simulink model "requirements"  (R2022a)
settings: Solver=VariableStepAuto  StartTime=0.0  StopTime=10.0  RelTol=1e-3
settings Model: Creator=aldra  LastModifiedBy=aldra
settings ModelReferenceCC: EnableRefExpFcnMdlSchedulingChecks=off
settings RTWCC: Description=Generic Real-Time Target

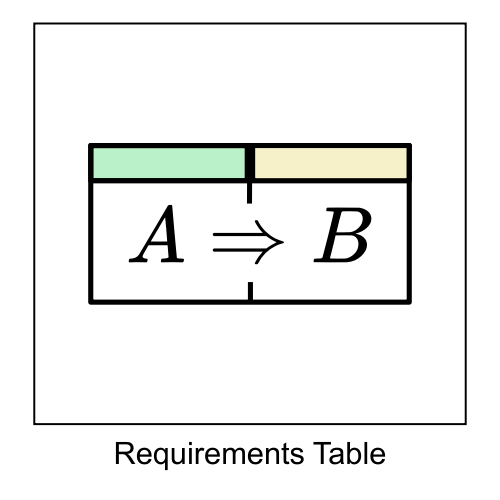
[thumbnail: Simulink's stored preview of the top-level diagram]
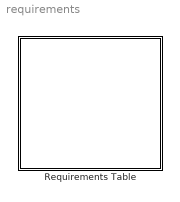
== system requirements ==
  Requirements Table : Requirements Table  TreatAsAtomicUnit=on

== stateflow chart requirements/Requirements Table ==
  (default) -> (junction 1073742735)
  (junction 1073742735) -> (junction 1073742736) : {
      | % SF_REQ_REV_07
      | }
  (junction 1073742736) -> (junction 1073742738) : {
      | % HEADER_ASSIGNMENTS
      |
      | }
  (junction 1073742738) -> (junction 1073742740) : {
      | % START_A_4
      | }
  (junction 1073742740) -> (junction 1073742742) : {
      | }
  (junction 1073742742) -> (junction 1073742744)
  (junction 1073742744) -> (junction 1073742746) : {
      | }
  (junction 1073742746) -> (junction 1073742748) : {
      | % END_A_4
      | }
  (junction 1073742748) -> (junction 1073742750) : {
      | % START_R_1
      | }
  (junction 1073742750) -> (junction 1073742752) : {
      | }
  (junction 1073742752) -> (junction 1073742754) : {
      |
      |
      | }
  (junction 1073742754) -> (junction 1073742756) : {
      | }
  (junction 1073742756) -> (junction 1073742758) : {
      | % START_R_7
      | }
  (junction 1073742758) -> (junction 1073742760) : {
      | }
  (junction 1073742760) -> (junction 1073742762)
  (junction 1073742762) -> (junction 1073742764) [order 1] : [(MODE.AOO == MODE)]
  (junction 1073742762) -> (junction 1073742770) [order 2]
  (junction 1073742764) -> (junction 1073742766) : {
      | reqtable_postcondition((USE_ATR_AMP == true), 'R:1.1');
      |
      |
      | }
  (junction 1073742766) -> (junction 1073742768) : {
      | }
  (junction 1073742768) -> (junction 1073742770)
  (junction 1073742770) -> (junction 1073742772)
  (junction 1073742772) -> (junction 1073742774) : {
      | % END_R_7
      | }
  (junction 1073742774) -> (junction 1073742776) : {
      | % START_R_10
      | }
  (junction 1073742776) -> (junction 1073742778) : {
      | }
  (junction 1073742778) -> (junction 1073742780)
  (junction 1073742780) -> (junction 1073742782) [order 1] : [(MODE.AOO == MODE)]
  (junction 1073742780) -> (junction 1073742788) [order 2]
  (junction 1073742782) -> (junction 1073742784) : {
      | reqtable_postcondition((OUTPUT_ATR == true), 'R:1.2');
      |
      |
      | }
  (junction 1073742784) -> (junction 1073742786) : {
      | }
  (junction 1073742786) -> (junction 1073742788)
  (junction 1073742788) -> (junction 1073742790)
  (junction 1073742790) -> (junction 1073742792) : {
      | % END_R_10
      | }
  (junction 1073742792) -> (junction 1073742794) : {
      | % START_R_40
      | }
  (junction 1073742794) -> (junction 1073742796) : {
      | }
  (junction 1073742796) -> (junction 1073742798) : {
      |
      |
      | }
  (junction 1073742798) -> (junction 1073742800) : {
      | }
  (junction 1073742800) -> (junction 1073742802) : {
      | % START_R_43
      | }
  (junction 1073742802) -> (junction 1073742804) : {
      | }
  (junction 1073742804) -> (junction 1073742806)
  (junction 1073742806) -> (junction 1073742808) [order 1] : [(DISCHARGE_ATR > 0)]
  (junction 1073742806) -> (junction 1073742814) [order 2]
  (junction 1073742808) -> (junction 1073742810) : {
      | reqtable_postcondition((PACE_CHARGE_CTRL == false), 'R:1.3.1');
      |
      |
      | }
  (junction 1073742810) -> (junction 1073742812) : {
      | }
  (junction 1073742812) -> (junction 1073742814)
  (junction 1073742814) -> (junction 1073742816)
  (junction 1073742816) -> (junction 1073742818) : {
      | % END_R_43
      | }
  (junction 1073742818) -> (junction 1073742820) : {
      | % START_R_46
      | }
  (junction 1073742820) -> (junction 1073742822) : {
      | }
  (junction 1073742822) -> (junction 1073742824)
  (junction 1073742824) -> (junction 1073742826) [order 1] : [(DISCHARGE_ATR > 0)]
  (junction 1073742824) -> (junction 1073742832) [order 2]
  (junction 1073742826) -> (junction 1073742828) : {
      | reqtable_postcondition((PACE_GND_CTRL == true), 'R:1.3.2');
      |
      |
      | }
  (junction 1073742828) -> (junction 1073742830) : {
      | }
  (junction 1073742830) -> (junction 1073742832)
  (junction 1073742832) -> (junction 1073742834)
  (junction 1073742834) -> (junction 1073742836) : {
      | % END_R_46
      | }
  (junction 1073742836) -> (junction 1073742838) : {
      | % START_R_49
      | }
  (junction 1073742838) -> (junction 1073742840) : {
      | }
  (junction 1073742840) -> (junction 1073742842)
  (junction 1073742842) -> (junction 1073742844) [order 1] : [(DISCHARGE_ATR > 0)]
  (junction 1073742842) -> (junction 1073742850) [order 2]
  (junction 1073742844) -> (junction 1073742846) : {
      | reqtable_postcondition((VENT_PACE_CTRL == false), 'R:1.3.3');
      |
      |
      | }
  (junction 1073742846) -> (junction 1073742848) : {
      | }
  (junction 1073742848) -> (junction 1073742850)
  (junction 1073742850) -> (junction 1073742852)
  (junction 1073742852) -> (junction 1073742854) : {
      | % END_R_49
      | }
  (junction 1073742854) -> (junction 1073742856) : {
      | % START_R_52
      | }
  (junction 1073742856) -> (junction 1073742858) : {
      | }
  (junction 1073742858) -> (junction 1073742860)
  (junction 1073742860) -> (junction 1073742862) [order 1] : [(DISCHARGE_ATR > 0)]
  (junction 1073742860) -> (junction 1073742868) [order 2]
  (junction 1073742862) -> (junction 1073742864) : {
      | reqtable_postcondition((VENT_GND_CTRL== false), 'R:1.3.4');
      |
      |
      | }
  (junction 1073742864) -> (junction 1073742866) : {
      | }
  (junction 1073742866) -> (junction 1073742868)
  (junction 1073742868) -> (junction 1073742870)
  (junction 1073742870) -> (junction 1073742872) : {
      | % END_R_52
      | }
  (junction 1073742872) -> (junction 1073742874) : {
      | % START_R_55
      | }
  (junction 1073742874) -> (junction 1073742876) : {
      | }
  (junction 1073742876) -> (junction 1073742878)
  (junction 1073742878) -> (junction 1073742880) [order 1] : [(DISCHARGE_ATR > 0)]
  (junction 1073742878) -> (junction 1073742886) [order 2]
  (junction 1073742880) -> (junction 1073742882) : {
      | reqtable_postcondition((ATR_GND_CTRL== false), 'R:1.3.5');
      |
      |
      | }
  (junction 1073742882) -> (junction 1073742884) : {
      | }
  (junction 1073742884) -> (junction 1073742886)
  (junction 1073742886) -> (junction 1073742888)
  (junction 1073742888) -> (junction 1073742890) : {
      | % END_R_55
      | }
  (junction 1073742890) -> (junction 1073742892) : {
      | % START_R_58
      | }
  (junction 1073742892) -> (junction 1073742894) : {
      | }
  (junction 1073742894) -> (junction 1073742896)
  (junction 1073742896) -> (junction 1073742898) [order 1] : [(DISCHARGE_ATR > 0)]
  (junction 1073742896) -> (junction 1073742904) [order 2]
  (junction 1073742898) -> (junction 1073742900) : {
      | reqtable_postcondition((ATR_PACE_CTRL == true), 'R:1.3.6');
      |
      |
      | }
  (junction 1073742900) -> (junction 1073742902) : {
      | }
  (junction 1073742902) -> (junction 1073742904)
  (junction 1073742904) -> (junction 1073742906)
  (junction 1073742906) -> (junction 1073742908) : {
      | % END_R_58
      | }
  (junction 1073742908) -> (junction 1073742910) : {
      | % START_R_61
      | }
  (junction 1073742910) -> (junction 1073742912) : {
      | }
  (junction 1073742912) -> (junction 1073742914)
  (junction 1073742914) -> (junction 1073742916) [order 1] : [(DISCHARGE_ATR > 0)]
  (junction 1073742914) -> (junction 1073742922) [order 2]
  (junction 1073742916) -> (junction 1073742918) : {
      | reqtable_postcondition((Z_VENT_CTRL == false), 'R:1.3.7');
      |
      |
      | }
  (junction 1073742918) -> (junction 1073742920) : {
      | }
  (junction 1073742920) -> (junction 1073742922)
  (junction 1073742922) -> (junction 1073742924)
  (junction 1073742924) -> (junction 1073742926) : {
      | % END_R_61
      | }
  (junction 1073742926) -> (junction 1073742928) : {
      | % START_R_64
      | }
  (junction 1073742928) -> (junction 1073742930) : {
      | }
  (junction 1073742930) -> (junction 1073742932)
  (junction 1073742932) -> (junction 1073742934) [order 1] : [(DISCHARGE_ATR > 0)]
  (junction 1073742932) -> (junction 1073742940) [order 2]
  (junction 1073742934) -> (junction 1073742936) : {
      | reqtable_postcondition((Z_ATR_CTRL == false), 'R:1.3.8');
      |
      |
      | }
  (junction 1073742936) -> (junction 1073742938) : {
      | }
  (junction 1073742938) -> (junction 1073742940)
  (junction 1073742940) -> (junction 1073742942)
  (junction 1073742942) -> (junction 1073742962) : {
      | % END_R_64
      | }
  (junction 1073742962) -> (junction 1073743289) : {
      | % START_R_97
      | }
  (junction 1073743289) -> (junction 1073743291) : {
      | }
  (junction 1073743291) -> (junction 1073743293)
  (junction 1073743293) -> (junction 1073743295) [order 1] : [(time > ATR_PULSE_WIDTH)]
  (junction 1073743293) -> (junction 1073743301) [order 2]
  (junction 1073743295) -> (junction 1073743297) : {
      | reqtable_postcondition((ATR_PACE_CTRL == false), 'R:1.3.9');
      |
      |
      | }
  (junction 1073743297) -> (junction 1073743299) : {
      | }
  (junction 1073743299) -> (junction 1073743301)
  (junction 1073743301) -> (junction 1073743303)
  (junction 1073743303) -> (junction 1073743389) : {
      | % END_R_97
      | }
  (junction 1073743389) -> (junction 1073743394) : {
      | % START_R_112
      | }
  (junction 1073743394) -> (junction 1073743396) : {
      | }
  (junction 1073743396) -> (junction 1073743398)
  (junction 1073743398) -> (junction 1073743400) [order 1] : [(time > ATR_PULSE_WIDTH)]
  (junction 1073743398) -> (junction 1073743406) [order 2]
  (junction 1073743400) -> (junction 1073743402) : {
      | reqtable_postcondition((ATR_GND_CTRL == true), 'R:1.3.10');
      |
      |
      | }
  (junction 1073743402) -> (junction 1073743404) : {
      | }
  (junction 1073743404) -> (junction 1073743406)
  (junction 1073743406) -> (junction 1073743408)
  (junction 1073743408) -> (junction 1073743431) : {
      | % END_R_112
      | }
  (junction 1073743431) -> (junction 1073743277) : {
      | % END_R_40
      | }
  (junction 1073743277) -> (junction 1073742966) : {
      | % END_R_1
      | }
  (junction 1073742966) -> (junction 1073742968) : {
      | % START_R_13
      | }
  (junction 1073742968) -> (junction 1073742970) : {
      | }
  (junction 1073742970) -> (junction 1073742972) : {
      |
      |
      | }
  (junction 1073742972) -> (junction 1073742974) : {
      | }
  (junction 1073742974) -> (junction 1073742976) : {
      | % START_R_16
      | }
  (junction 1073742976) -> (junction 1073742978) : {
      | }
  (junction 1073742978) -> (junction 1073742980)
  (junction 1073742980) -> (junction 1073742982) [order 1] : [(MODE.VOO == MODE2)]
  (junction 1073742980) -> (junction 1073742988) [order 2]
  (junction 1073742982) -> (junction 1073742984) : {
      | reqtable_postcondition((USE_ATR_AMP == false), 'R:2.1');
      |
      |
      | }
  (junction 1073742984) -> (junction 1073742986) : {
      | }
  (junction 1073742986) -> (junction 1073742988)
  (junction 1073742988) -> (junction 1073742990)
  (junction 1073742990) -> (junction 1073742992) : {
      | % END_R_16
      | }
  (junction 1073742992) -> (junction 1073742994) : {
      | % START_R_19
      | }
  (junction 1073742994) -> (junction 1073742996) : {
      | }
  (junction 1073742996) -> (junction 1073742998)
  (junction 1073742998) -> (junction 1073743000) [order 1] : [(MODE.VOO == MODE2)]
  (junction 1073742998) -> (junction 1073743006) [order 2]
  (junction 1073743000) -> (junction 1073743002) : {
      | reqtable_postcondition((OUTPUT_VENT == true), 'R:2.2');
      |
      |
      | }
  (junction 1073743002) -> (junction 1073743004) : {
      | }
  (junction 1073743004) -> (junction 1073743006)
  (junction 1073743006) -> (junction 1073743008)
  (junction 1073743008) -> (junction 1073743010) : {
      | % END_R_19
      | }
  (junction 1073743010) -> (junction 1073743790) : {
      | % START_R_166
      | }
  (junction 1073743790) -> (junction 1073743792) : {
      | }
  (junction 1073743792) -> (junction 1073743794) : {
      |
      |
      | }
  (junction 1073743794) -> (junction 1073743796) : {
      | }
  (junction 1073743796) -> (junction 1073743798) : {
      | % START_R_169
      | }
  (junction 1073743798) -> (junction 1073743800) : {
      | }
  (junction 1073743800) -> (junction 1073743802)
  (junction 1073743802) -> (junction 1073743804) [order 1] : [(DISCHARGE_VENT > 0)]
  (junction 1073743802) -> (junction 1073743810) [order 2]
  (junction 1073743804) -> (junction 1073743806) : {
      | reqtable_postcondition((PACE_CHARGE_CTRL == false), 'R:2.3.1');
      |
      |
      | }
  (junction 1073743806) -> (junction 1073743808) : {
      | }
  (junction 1073743808) -> (junction 1073743810)
  (junction 1073743810) -> (junction 1073743812)
  (junction 1073743812) -> (junction 1073743814) : {
      | % END_R_169
      | }
  (junction 1073743814) -> (junction 1073743816) : {
      | % START_R_172
      | }
  (junction 1073743816) -> (junction 1073743818) : {
      | }
  (junction 1073743818) -> (junction 1073743820)
  (junction 1073743820) -> (junction 1073743822) [order 1] : [(DISCHARGE_VENT > 0)]
  (junction 1073743820) -> (junction 1073743828) [order 2]
  (junction 1073743822) -> (junction 1073743824) : {
      | reqtable_postcondition((PACE_GND_CTRL == true), 'R:2.3.2');
      |
      |
      | }
  (junction 1073743824) -> (junction 1073743826) : {
      | }
  (junction 1073743826) -> (junction 1073743828)
  (junction 1073743828) -> (junction 1073743830)
  (junction 1073743830) -> (junction 1073743832) : {
      | % END_R_172
      | }
  (junction 1073743832) -> (junction 1073743834) : {
      | % START_R_175
      | }
  (junction 1073743834) -> (junction 1073743836) : {
      | }
  (junction 1073743836) -> (junction 1073743838)
  (junction 1073743838) -> (junction 1073743840) [order 1] : [(DISCHARGE_VENT > 0)]
  (junction 1073743838) -> (junction 1073743846) [order 2]
  (junction 1073743840) -> (junction 1073743842) : {
      | reqtable_postcondition((VENT_PACE_CTRL == true), 'R:2.3.3');
      |
      |
      | }
  (junction 1073743842) -> (junction 1073743844) : {
      | }
  (junction 1073743844) -> (junction 1073743846)
  (junction 1073743846) -> (junction 1073743848)
  (junction 1073743848) -> (junction 1073743850) : {
      | % END_R_175
      | }
  (junction 1073743850) -> (junction 1073743852) : {
      | % START_R_178
      | }
  (junction 1073743852) -> (junction 1073743854) : {
      | }
  (junction 1073743854) -> (junction 1073743856)
  (junction 1073743856) -> (junction 1073743858) [order 1] : [(DISCHARGE_VENT > 0)]
  (junction 1073743856) -> (junction 1073743864) [order 2]
  (junction 1073743858) -> (junction 1073743860) : {
      | reqtable_postcondition((VENT_GND_CTRL== false), 'R:2.3.4');
      |
      |
      | }
  (junction 1073743860) -> (junction 1073743862) : {
      | }
  (junction 1073743862) -> (junction 1073743864)
  (junction 1073743864) -> (junction 1073743866)
  (junction 1073743866) -> (junction 1073743868) : {
      | % END_R_178
      | }
  (junction 1073743868) -> (junction 1073743870) : {
      | % START_R_181
      | }
  (junction 1073743870) -> (junction 1073743872) : {
      | }
  (junction 1073743872) -> (junction 1073743874)
  (junction 1073743874) -> (junction 1073743876) [order 1] : [(DISCHARGE_VENT > 0)]
  (junction 1073743874) -> (junction 1073743882) [order 2]
  (junction 1073743876) -> (junction 1073743878) : {
      | reqtable_postcondition((ATR_GND_CTRL== false), 'R:2.3.5');
      |
      |
      | }
  (junction 1073743878) -> (junction 1073743880) : {
      | }
  (junction 1073743880) -> (junction 1073743882)
  (junction 1073743882) -> (junction 1073743884)
  (junction 1073743884) -> (junction 1073743886) : {
      | % END_R_181
      | }
  (junction 1073743886) -> (junction 1073743888) : {
      | % START_R_184
      | }
  (junction 1073743888) -> (junction 1073743890) : {
      | }
  (junction 1073743890) -> (junction 1073743892)
  (junction 1073743892) -> (junction 1073743894) [order 1] : [(DISCHARGE_VENT > 0)]
  (junction 1073743892) -> (junction 1073743900) [order 2]
  (junction 1073743894) -> (junction 1073743896) : {
      | reqtable_postcondition((ATR_PACE_CTRL == false), 'R:2.3.6');
      |
      |
      | }
  (junction 1073743896) -> (junction 1073743898) : {
      | }
  (junction 1073743898) -> (junction 1073743900)
  (junction 1073743900) -> (junction 1073743902)
  (junction 1073743902) -> (junction 1073743904) : {
      | % END_R_184
      | }
  (junction 1073743904) -> (junction 1073743906) : {
      | % START_R_187
      | }
  (junction 1073743906) -> (junction 1073743908) : {
      | }
  (junction 1073743908) -> (junction 1073743910)
  (junction 1073743910) -> (junction 1073743912) [order 1] : [(DISCHARGE_VENT > 0)]
  (junction 1073743910) -> (junction 1073743918) [order 2]
  (junction 1073743912) -> (junction 1073743914) : {
      | reqtable_postcondition((Z_VENT_CTRL == false), 'R:2.3.7');
      |
      |
      | }
  (junction 1073743914) -> (junction 1073743916) : {
      | }
  (junction 1073743916) -> (junction 1073743918)
  (junction 1073743918) -> (junction 1073743920)
  (junction 1073743920) -> (junction 1073743922) : {
      | % END_R_187
      | }
  (junction 1073743922) -> (junction 1073743924) : {
      | % START_R_190
      | }
  (junction 1073743924) -> (junction 1073743926) : {
      | }
  (junction 1073743926) -> (junction 1073743928)
  (junction 1073743928) -> (junction 1073743930) [order 1] : [(DISCHARGE_VENT > 0)]
  (junction 1073743928) -> (junction 1073743936) [order 2]
  (junction 1073743930) -> (junction 1073743932) : {
      | reqtable_postcondition((Z_ATR_CTRL == false), 'R:2.3.8');
      |
      |
      | }
  (junction 1073743932) -> (junction 1073743934) : {
      | }
  (junction 1073743934) -> (junction 1073743936)
  (junction 1073743936) -> (junction 1073743938)
  (junction 1073743938) -> (junction 1073743940) : {
      | % END_R_190
      | }
  (junction 1073743940) -> (junction 1073743942) : {
      | % START_R_193
      | }
  (junction 1073743942) -> (junction 1073743944) : {
      | }
  (junction 1073743944) -> (junction 1073743946)
  (junction 1073743946) -> (junction 1073743948) [order 1] : [(time > VENT_PULSE_WIDTH)]
  (junction 1073743946) -> (junction 1073743954) [order 2]
  (junction 1073743948) -> (junction 1073743950) : {
      | reqtable_postcondition((VENT_PACE_CTRL == false), 'R:2.3.9');
      |
      |
      | }
  (junction 1073743950) -> (junction 1073743952) : {
      | }
  (junction 1073743952) -> (junction 1073743954)
  (junction 1073743954) -> (junction 1073743956)
  (junction 1073743956) -> (junction 1073743958) : {
      | % END_R_193
      | }
  (junction 1073743958) -> (junction 1073743960) : {
      | % START_R_196
      | }
  (junction 1073743960) -> (junction 1073743962) : {
      | }
  (junction 1073743962) -> (junction 1073743964)
  (junction 1073743964) -> (junction 1073743966) [order 1] : [(time > VENT_PULSE_WIDTH)]
  (junction 1073743964) -> (junction 1073743972) [order 2]
  (junction 1073743966) -> (junction 1073743968) : {
      | reqtable_postcondition((VENT_GND_CTRL == true), 'R:2.3.10');
      |
      |
      | }
  (junction 1073743968) -> (junction 1073743970) : {
      | }
  (junction 1073743970) -> (junction 1073743972)
  (junction 1073743972) -> (junction 1073743974)
  (junction 1073743974) -> (junction 1073743976) : {
      | % END_R_196
      | }
  (junction 1073743976) -> (junction 1073743978) : {
      | % END_R_166
      | }
  (junction 1073743978) -> (junction 1073743012) : {
      | % END_R_13
      | }
  (junction 1073743012) -> (junction 1073743014) : {
      | % START_R_22
      | }
  (junction 1073743014) -> (junction 1073743016) : {
      | }
  (junction 1073743016) -> (junction 1073743018) : {
      |
      |
      | }
  (junction 1073743018) -> (junction 1073743020) : {
      | }
  (junction 1073743020) -> (junction 1073743022) : {
      | % START_R_25
      | }
  (junction 1073743022) -> (junction 1073743024) : {
      | }
  (junction 1073743024) -> (junction 1073743026)
  (junction 1073743026) -> (junction 1073743028) [order 1] : [(MODE.AAI == MODE1)]
  (junction 1073743026) -> (junction 1073743034) [order 2]
  (junction 1073743028) -> (junction 1073743030) : {
      | reqtable_postcondition((USE_ATR_AMP == true), 'R:3.1');
      |
      |
      | }
  (junction 1073743030) -> (junction 1073743032) : {
      | }
  (junction 1073743032) -> (junction 1073743034)
  (junction 1073743034) -> (junction 1073743036)
  (junction 1073743036) -> (junction 1073743038) : {
      | % END_R_25
      | }
  (junction 1073743038) -> (junction 1073743479) : {
      | % START_R_28
      | }
  (junction 1073743479) -> (junction 1073743481) : {
      | }
  (junction 1073743481) -> (junction 1073743483)
  (junction 1073743483) -> (junction 1073743485) [order 1] : [(MODE.AAI == MODE1)]
  (junction 1073743483) -> (junction 1073743491) [order 2]
  (junction 1073743485) -> (junction 1073743487) : {
      | reqtable_postcondition((OUTPUT_ATR == true), 'R:3.2');
      |
      |
      | }
  (junction 1073743487) -> (junction 1073743489) : {
      | }
  (junction 1073743489) -> (junction 1073743491)
  (junction 1073743491) -> (junction 1073743493)
  (junction 1073743493) -> (junction 1073743495) : {
      | % END_R_28
      | }
  (junction 1073743495) -> (junction 1073743512) : {
      | % START_R_124
      | }
  (junction 1073743512) -> (junction 1073743514) : {
      | }
  (junction 1073743514) -> (junction 1073743516) : {
      |
      |
      | }
  (junction 1073743516) -> (junction 1073743518) : {
      | }
  (junction 1073743518) -> (junction 1073743534) : {
      | % START_R_127
      | }
  (junction 1073743534) -> (junction 1073743536) : {
      | }
  (junction 1073743536) -> (junction 1073743538)
  (junction 1073743538) -> (junction 1073743540) [order 1] : [(NATRUAL_WAVE == true)]
  (junction 1073743538) -> (junction 1073743546) [order 2]
  (junction 1073743540) -> (junction 1073743542) : {
      | output = 0
      |
      | }
  (junction 1073743542) -> (junction 1073743544) : {
      | }
  (junction 1073743544) -> (junction 1073743546)
  (junction 1073743546) -> (junction 1073743548)
  (junction 1073743548) -> (junction 1073743550) : {
      | % END_R_127
      | }
  (junction 1073743550) -> (junction 1073743567) : {
      | % START_R_130
      | }
  (junction 1073743567) -> (junction 1073743569) : {
      | }
  (junction 1073743569) -> (junction 1073743571)
  (junction 1073743571) -> (junction 1073743573) [order 1] : [(NATURAL_WAVE == false)]
  (junction 1073743571) -> (junction 1073743579) [order 2]
  (junction 1073743573) -> (junction 1073743575) : {
      | output = 1
      |
      | }
  (junction 1073743575) -> (junction 1073743577) : {
      | }
  (junction 1073743577) -> (junction 1073743579)
  (junction 1073743579) -> (junction 1073743581)
  (junction 1073743581) -> (junction 1073743583) : {
      | % END_R_130
      | }
  (junction 1073743583) -> (junction 1073743588) : {
      | % START_R_133
      | }
  (junction 1073743588) -> (junction 1073743590) : {
      | }
  (junction 1073743590) -> (junction 1073743592) : {
      |
      |
      | }
  (junction 1073743592) -> (junction 1073743594) : {
      | }
  (junction 1073743594) -> (junction 1073743596) : {
      | % START_R_136
      | }
  (junction 1073743596) -> (junction 1073743598) : {
      | }
  (junction 1073743598) -> (junction 1073743600)
  (junction 1073743600) -> (junction 1073743602) [order 1] : [(DISCHARGE_ATR == true)]
  (junction 1073743600) -> (junction 1073743608) [order 2]
  (junction 1073743602) -> (junction 1073743604) : {
      | reqtable_postcondition((PACE_CHARGE_CTRL == false), 'R:3.3.3.1');
      |
      |
      | }
  (junction 1073743604) -> (junction 1073743606) : {
      | }
  (junction 1073743606) -> (junction 1073743608)
  (junction 1073743608) -> (junction 1073743610)
  (junction 1073743610) -> (junction 1073743612) : {
      | % END_R_136
      | }
  (junction 1073743612) -> (junction 1073743614) : {
      | % START_R_139
      | }
  (junction 1073743614) -> (junction 1073743616) : {
      | }
  (junction 1073743616) -> (junction 1073743618)
  (junction 1073743618) -> (junction 1073743620) [order 1] : [(DISCHARGE_ATR == true)]
  (junction 1073743618) -> (junction 1073743626) [order 2]
  (junction 1073743620) -> (junction 1073743622) : {
      | reqtable_postcondition((PACE_GND_CTRL == false), 'R:3.3.3.2');
      |
      |
      | }
  (junction 1073743622) -> (junction 1073743624) : {
      | }
  (junction 1073743624) -> (junction 1073743626)
  (junction 1073743626) -> (junction 1073743628)
  (junction 1073743628) -> (junction 1073743630) : {
      | % END_R_139
      | }
  (junction 1073743630) -> (junction 1073743632) : {
      | % START_R_142
      | }
  (junction 1073743632) -> (junction 1073743634) : {
      | }
  (junction 1073743634) -> (junction 1073743636)
  (junction 1073743636) -> (junction 1073743638) [order 1] : [(DISCHARGE_ATR == true)]
  (junction 1073743636) -> (junction 1073743644) [order 2]
  (junction 1073743638) -> (junction 1073743640) : {
      | reqtable_postcondition((VENT_PACE_CTRL == false), 'R:3.3.3.3');
      |
      |
      | }
  (junction 1073743640) -> (junction 1073743642) : {
      | }
  (junction 1073743642) -> (junction 1073743644)
  (junction 1073743644) -> (junction 1073743646)
  (junction 1073743646) -> (junction 1073743648) : {
      | % END_R_142
      | }
  (junction 1073743648) -> (junction 1073743650) : {
      | % START_R_145
      | }
  (junction 1073743650) -> (junction 1073743652) : {
      | }
  (junction 1073743652) -> (junction 1073743654)
  (junction 1073743654) -> (junction 1073743656) [order 1] : [(DISCHARGE_ATR == true)]
  (junction 1073743654) -> (junction 1073743662) [order 2]
  (junction 1073743656) -> (junction 1073743658) : {
      | reqtable_postcondition((VENT_GND_CTRL== false), 'R:3.3.3.4');
      |
      |
      | }
  (junction 1073743658) -> (junction 1073743660) : {
      | }
  (junction 1073743660) -> (junction 1073743662)
  (junction 1073743662) -> (junction 1073743664)
  (junction 1073743664) -> (junction 1073743666) : {
      | % END_R_145
      | }
  (junction 1073743666) -> (junction 1073743668) : {
      | % START_R_148
      | }
  (junction 1073743668) -> (junction 1073743670) : {
      | }
  (junction 1073743670) -> (junction 1073743672)
  (junction 1073743672) -> (junction 1073743674) [order 1] : [(DISCHARGE_ATR == true)]
  (junction 1073743672) -> (junction 1073743680) [order 2]
  (junction 1073743674) -> (junction 1073743676) : {
      | reqtable_postcondition((ATR_GND_CTRL== false), 'R:3.3.3.5');
      |
      |
      | }
  (junction 1073743676) -> (junction 1073743678) : {
      | }
  (junction 1073743678) -> (junction 1073743680)
  (junction 1073743680) -> (junction 1073743682)
  (junction 1073743682) -> (junction 1073743684) : {
      | % END_R_148
      | }
  (junction 1073743684) -> (junction 1073743686) : {
      | % START_R_151
      | }
  (junction 1073743686) -> (junction 1073743688) : {
      | }
  (junction 1073743688) -> (junction 1073743690)
  (junction 1073743690) -> (junction 1073743692) [order 1] : [(DISCHARGE_ATR == true)]
  (junction 1073743690) -> (junction 1073743698) [order 2]
  (junction 1073743692) -> (junction 1073743694) : {
      | reqtable_postcondition((ATR_PACE_CTRL == true), 'R:3.3.3.6');
      |
      |
      | }
  (junction 1073743694) -> (junction 1073743696) : {
      | }
  (junction 1073743696) -> (junction 1073743698)
  (junction 1073743698) -> (junction 1073743700)
  (junction 1073743700) -> (junction 1073743702) : {
      | % END_R_151
      | }
  (junction 1073743702) -> (junction 1073743704) : {
      | % START_R_154
      | }
  (junction 1073743704) -> (junction 1073743706) : {
      | }
  (junction 1073743706) -> (junction 1073743708)
  (junction 1073743708) -> (junction 1073743710) [order 1] : [(DISCHARGE_ATR == true)]
  (junction 1073743708) -> (junction 1073743716) [order 2]
  (junction 1073743710) -> (junction 1073743712) : {
      | reqtable_postcondition((Z_VENT_CTRL == false), 'R:3.3.3.7');
      |
      |
      | }
  (junction 1073743712) -> (junction 1073743714) : {
      | }
  (junction 1073743714) -> (junction 1073743716)
  (junction 1073743716) -> (junction 1073743718)
  (junction 1073743718) -> (junction 1073743720) : {
      | % END_R_154
      | }
  (junction 1073743720) -> (junction 1073743722) : {
      | % START_R_157
      | }
  (junction 1073743722) -> (junction 1073743724) : {
      | }
  (junction 1073743724) -> (junction 1073743726)
  (junction 1073743726) -> (junction 1073743728) [order 1] : [(DISCHARGE_ATR == true)]
  (junction 1073743726) -> (junction 1073743734) [order 2]
  (junction 1073743728) -> (junction 1073743730) : {
      | reqtable_postcondition((Z_ATR_CTRL == true), 'R:3.3.3.8');
      |
      |
      | }
  (junction 1073743730) -> (junction 1073743732) : {
      | }
  (junction 1073743732) -> (junction 1073743734)
  (junction 1073743734) -> (junction 1073743736)
  (junction 1073743736) -> (junction 1073743738) : {
      | % END_R_157
      | }
  (junction 1073743738) -> (junction 1073743740) : {
      | % START_R_160
      | }
  (junction 1073743740) -> (junction 1073743742) : {
      | }
  (junction 1073743742) -> (junction 1073743744)
  (junction 1073743744) -> (junction 1073743746) [order 1] : [(time > ATR_PULSE_WIDTH)]
  (junction 1073743744) -> (junction 1073743752) [order 2]
  (junction 1073743746) -> (junction 1073743748) : {
      | reqtable_postcondition((ATR_PACE_CTRL == false), 'R:3.3.3.9');
      |
      |
      | }
  (junction 1073743748) -> (junction 1073743750) : {
      | }
  (junction 1073743750) -> (junction 1073743752)
  (junction 1073743752) -> (junction 1073743754)
  (junction 1073743754) -> (junction 1073743756) : {
      | % END_R_160
      | }
  (junction 1073743756) -> (junction 1073743758) : {
      | % START_R_163
      | }
  (junction 1073743758) -> (junction 1073743760) : {
      | }
  (junction 1073743760) -> (junction 1073743762)
  (junction 1073743762) -> (junction 1073743764) [order 1] : [(time > ATR_PULSE_WIDTH)]
  (junction 1073743762) -> (junction 1073743770) [order 2]
  (junction 1073743764) -> (junction 1073743766) : {
      | reqtable_postcondition((ATR_GND_CTRL == true), 'R:3.3.3.10');
      |
      |
      | }
  (junction 1073743766) -> (junction 1073743768) : {
      | }
  (junction 1073743768) -> (junction 1073743770)
  (junction 1073743770) -> (junction 1073743772)
  (junction 1073743772) -> (junction 1073743774) : {
      | % END_R_163
      | }
  (junction 1073743774) -> (junction 1073743776) : {
      | % END_R_133
      | }
  (junction 1073743776) -> (junction 1073743530) : {
      | % END_R_124
      | }
  (junction 1073743530) -> (junction 1073743058) : {
      | % END_R_22
      | }
  (junction 1073743058) -> (junction 1073743060) : {
      | % START_R_31
      | }
  (junction 1073743060) -> (junction 1073743062) : {
      | }
  (junction 1073743062) -> (junction 1073743064) : {
      |
      |
      | }
  (junction 1073743064) -> (junction 1073743066) : {
      | }
  (junction 1073743066) -> (junction 1073743068) : {
      | % START_R_34
      | }
  (junction 1073743068) -> (junction 1073743070) : {
      | }
  (junction 1073743070) -> (junction 1073743072)
  (junction 1073743072) -> (junction 1073743074) [order 1] : [(MODE.VVI == MODE3)]
  (junction 1073743072) -> (junction 1073743080) [order 2]
  (junction 1073743074) -> (junction 1073743076) : {
      | reqtable_postcondition((USE_ATR_AMP == false), 'R:4.1');
      |
      |
      | }
  (junction 1073743076) -> (junction 1073743078) : {
      | }
  (junction 1073743078) -> (junction 1073743080)
  (junction 1073743080) -> (junction 1073743082)
  (junction 1073743082) -> (junction 1073743084) : {
      | % END_R_34
      | }
  (junction 1073743084) -> (junction 1073743086) : {
      | % START_R_37
      | }
  (junction 1073743086) -> (junction 1073743088) : {
      | }
  (junction 1073743088) -> (junction 1073743090)
  (junction 1073743090) -> (junction 1073743092) [order 1] : [(MODE.VVI== MODE3)]
  (junction 1073743090) -> (junction 1073743098) [order 2]
  (junction 1073743092) -> (junction 1073743094) : {
      | reqtable_postcondition((OUTPUT_VENT == true), 'R:4.2');
      |
      |
      | }
  (junction 1073743094) -> (junction 1073743096) : {
      | }
  (junction 1073743096) -> (junction 1073743098)
  (junction 1073743098) -> (junction 1073743100)
  (junction 1073743100) -> (junction 1073743102) : {
      | % END_R_37
      | }
  (junction 1073743102) -> (junction 1073744004) : {
      | % START_R_199
      | }
  (junction 1073744004) -> (junction 1073744006) : {
      | }
  (junction 1073744006) -> (junction 1073744008) : {
      |
      |
      | }
  (junction 1073744008) -> (junction 1073744020) : {
      | }
  (junction 1073744020) -> (junction 1073744026) : {
      | % START_R_205
      | }
  (junction 1073744026) -> (junction 1073744028) : {
      | }
  (junction 1073744028) -> (junction 1073744030)
  (junction 1073744030) -> (junction 1073744032) [order 1] : [(NATRUAL_WAVE == true)]
  (junction 1073744030) -> (junction 1073744038) [order 2]
  (junction 1073744032) -> (junction 1073744034) : {
      | output = 0
      |
      | }
  (junction 1073744034) -> (junction 1073744036) : {
      | }
  (junction 1073744036) -> (junction 1073744038)
  (junction 1073744038) -> (junction 1073744040)
  (junction 1073744040) -> (junction 1073744042) : {
      | % END_R_205
      | }
  (junction 1073744042) -> (junction 1073744047) : {
      | % START_R_208
      | }
  (junction 1073744047) -> (junction 1073744049) : {
      | }
  (junction 1073744049) -> (junction 1073744051)
  (junction 1073744051) -> (junction 1073744053) [order 1] : [(NATURAL_WAVE == false)]
  (junction 1073744051) -> (junction 1073744059) [order 2]
  (junction 1073744053) -> (junction 1073744055) : {
      | output = 1
      |
      | }
  (junction 1073744055) -> (junction 1073744057) : {
      | }
  (junction 1073744057) -> (junction 1073744059)
  (junction 1073744059) -> (junction 1073744061)
  (junction 1073744061) -> (junction 1073744063) : {
      | % END_R_208
      | }
  (junction 1073744063) -> (junction 1073744068) : {
      | % START_R_211
      | }
  (junction 1073744068) -> (junction 1073744070) : {
      | }
  (junction 1073744070) -> (junction 1073744072) : {
      |
      |
      | }
  (junction 1073744072) -> (junction 1073744074) : {
      | }
  (junction 1073744074) -> (junction 1073744076) : {
      | % START_R_214
      | }
  (junction 1073744076) -> (junction 1073744078) : {
      | }
  (junction 1073744078) -> (junction 1073744080)
  (junction 1073744080) -> (junction 1073744082) [order 1] : [(DISCHARGE_VENT > 0)]
  (junction 1073744080) -> (junction 1073744088) [order 2]
  (junction 1073744082) -> (junction 1073744084) : {
      | reqtable_postcondition((PACE_CHARGE_CTRL == false), 'R:4.3.3.1');
      |
      |
      | }
  (junction 1073744084) -> (junction 1073744086) : {
      | }
  (junction 1073744086) -> (junction 1073744088)
  (junction 1073744088) -> (junction 1073744090)
  (junction 1073744090) -> (junction 1073744092) : {
      | % END_R_214
      | }
  (junction 1073744092) -> (junction 1073744094) : {
      | % START_R_217
      | }
  (junction 1073744094) -> (junction 1073744096) : {
      | }
  (junction 1073744096) -> (junction 1073744098)
  (junction 1073744098) -> (junction 1073744100) [order 1] : [(DISCHARGE_VENT > 0)]
  (junction 1073744098) -> (junction 1073744106) [order 2]
  (junction 1073744100) -> (junction 1073744102) : {
      | reqtable_postcondition((PACE_GND_CTRL == true), 'R:4.3.3.2');
      |
      |
      | }
  (junction 1073744102) -> (junction 1073744104) : {
      | }
  (junction 1073744104) -> (junction 1073744106)
  (junction 1073744106) -> (junction 1073744108)
  (junction 1073744108) -> (junction 1073744110) : {
      | % END_R_217
      | }
  (junction 1073744110) -> (junction 1073744112) : {
      | % START_R_220
      | }
  (junction 1073744112) -> (junction 1073744114) : {
      | }
  (junction 1073744114) -> (junction 1073744116)
  (junction 1073744116) -> (junction 1073744118) [order 1] : [(DISCHARGE_VENT > 0)]
  (junction 1073744116) -> (junction 1073744124) [order 2]
  (junction 1073744118) -> (junction 1073744120) : {
      | reqtable_postcondition((VENT_PACE_CTRL == true), 'R:4.3.3.3');
      |
      |
      | }
  (junction 1073744120) -> (junction 1073744122) : {
      | }
  (junction 1073744122) -> (junction 1073744124)
  (junction 1073744124) -> (junction 1073744126)
  (junction 1073744126) -> (junction 1073744128) : {
      | % END_R_220
      | }
  (junction 1073744128) -> (junction 1073744130) : {
      | % START_R_223
      | }
  (junction 1073744130) -> (junction 1073744132) : {
      | }
  (junction 1073744132) -> (junction 1073744134)
  (junction 1073744134) -> (junction 1073744136) [order 1] : [(DISCHARGE_VENT > 0)]
  (junction 1073744134) -> (junction 1073744142) [order 2]
  (junction 1073744136) -> (junction 1073744138) : {
      | reqtable_postcondition((VENT_GND_CTRL== false), 'R:4.3.3.4');
      |
      |
      | }
  (junction 1073744138) -> (junction 1073744140) : {
      | }
  (junction 1073744140) -> (junction 1073744142)
  (junction 1073744142) -> (junction 1073744144)
  (junction 1073744144) -> (junction 1073744146) : {
      | % END_R_223
      | }
  (junction 1073744146) -> (junction 1073744148) : {
      | % START_R_226
      | }
  (junction 1073744148) -> (junction 1073744150) : {
      | }
  (junction 1073744150) -> (junction 1073744152)
  (junction 1073744152) -> (junction 1073744154) [order 1] : [(DISCHARGE_VENT > 0)]
  (junction 1073744152) -> (junction 1073744160) [order 2]
  (junction 1073744154) -> (junction 1073744156) : {
      | reqtable_postcondition((ATR_GND_CTRL== false), 'R:4.3.3.5');
      |
      |
      | }
  (junction 1073744156) -> (junction 1073744158) : {
      | }
  (junction 1073744158) -> (junction 1073744160)
  (junction 1073744160) -> (junction 1073744162)
  (junction 1073744162) -> (junction 1073744164) : {
      | % END_R_226
      | }
  (junction 1073744164) -> (junction 1073744166) : {
      | % START_R_229
      | }
  (junction 1073744166) -> (junction 1073744168) : {
      | }
  (junction 1073744168) -> (junction 1073744170)
  (junction 1073744170) -> (junction 1073744172) [order 1] : [(DISCHARGE_VENT > 0)]
  (junction 1073744170) -> (junction 1073744178) [order 2]
  (junction 1073744172) -> (junction 1073744174) : {
      | reqtable_postcondition((ATR_PACE_CTRL == false), 'R:4.3.3.6');
      |
      |
      | }
  (junction 1073744174) -> (junction 1073744176) : {
      | }
  (junction 1073744176) -> (junction 1073744178)
  (junction 1073744178) -> (junction 1073744180)
  (junction 1073744180) -> (junction 1073744182) : {
      | % END_R_229
      | }
  (junction 1073744182) -> (junction 1073744184) : {
      | % START_R_232
      | }
  (junction 1073744184) -> (junction 1073744186) : {
      | }
  (junction 1073744186) -> (junction 1073744188)
  (junction 1073744188) -> (junction 1073744190) [order 1] : [(DISCHARGE_VENT > 0)]
  (junction 1073744188) -> (junction 1073744196) [order 2]
  (junction 1073744190) -> (junction 1073744192) : {
      | reqtable_postcondition((Z_VENT_CTRL == false), 'R:4.3.3.7');
      |
      |
      | }
  (junction 1073744192) -> (junction 1073744194) : {
      | }
  (junction 1073744194) -> (junction 1073744196)
  (junction 1073744196) -> (junction 1073744198)
  (junction 1073744198) -> (junction 1073744200) : {
      | % END_R_232
      | }
  (junction 1073744200) -> (junction 1073744202) : {
      | % START_R_235
      | }
  (junction 1073744202) -> (junction 1073744204) : {
      | }
  (junction 1073744204) -> (junction 1073744206)
  (junction 1073744206) -> (junction 1073744208) [order 1] : [(DISCHARGE_VENT > 0)]
  (junction 1073744206) -> (junction 1073744214) [order 2]
  (junction 1073744208) -> (junction 1073744210) : {
      | reqtable_postcondition((Z_ATR_CTRL == false), 'R:4.3.3.8');
      |
      |
      | }
  (junction 1073744210) -> (junction 1073744212) : {
      | }
  (junction 1073744212) -> (junction 1073744214)
  (junction 1073744214) -> (junction 1073744216)
  (junction 1073744216) -> (junction 1073744218) : {
      | % END_R_235
      | }
  (junction 1073744218) -> (junction 1073744220) : {
      | % START_R_238
      | }
  (junction 1073744220) -> (junction 1073744222) : {
      | }
  (junction 1073744222) -> (junction 1073744224)
  (junction 1073744224) -> (junction 1073744226) [order 1] : [(time > VENT_PULSE_WIDTH)]
  (junction 1073744224) -> (junction 1073744232) [order 2]
  (junction 1073744226) -> (junction 1073744228) : {
      | reqtable_postcondition((VENT_PACE_CTRL == false), 'R:4.3.3.9');
      |
      |
      | }
  (junction 1073744228) -> (junction 1073744230) : {
      | }
  (junction 1073744230) -> (junction 1073744232)
  (junction 1073744232) -> (junction 1073744234)
  (junction 1073744234) -> (junction 1073744236) : {
      | % END_R_238
      | }
  (junction 1073744236) -> (junction 1073744238) : {
      | % START_R_241
      | }
  (junction 1073744238) -> (junction 1073744240) : {
      | }
  (junction 1073744240) -> (junction 1073744242)
  (junction 1073744242) -> (junction 1073744244) [order 1] : [(time > VENT_PULSE_WIDTH)]
  (junction 1073744242) -> (junction 1073744250) [order 2]
  (junction 1073744244) -> (junction 1073744246) : {
      | reqtable_postcondition((VENT_GND_CTRL == true), 'R:4.3.3.10');
      |
      |
      | }
  (junction 1073744246) -> (junction 1073744248) : {
      | }
  (junction 1073744248) -> (junction 1073744250)
  (junction 1073744250) -> (junction 1073744252)
  (junction 1073744252) -> (junction 1073744254) : {
      | % END_R_241
      | }
  (junction 1073744254) -> (junction 1073744256) : {
      | % END_R_211
      | }
  (junction 1073744256) -> (junction 1073744022) : {
      | % END_R_199
      | }
  (junction 1073744022) -> (junction 1073743104) : {
      | % END_R_31
      | }
